simulink model "MSFartoystyringSCtuning"  (R2017b)
settings: Solver=ode45  StartTime=tstart  StopTime=tstop  RelTol=1e-3  EnableMultiTasking=on
values from neighbouring files (symbols this model uses):
  c = 1    [SCtune.m]
  p0 = zeros(2,1)    [SCtune.m]
  psi0 = 0    [SCtune.m]
  r0 = 0    [SCtune.m]
  tsamp = 10    [SCtune.m]
  v0 = [3 0]'    [SCtune.m]
undefined symbols (not defined in the file or in its folder): delta_max, heading_controller, K_iu, K_psi, K_pu, K_u, L_pp, msfartoystyring, n_max, speed_controller, T_psi, T_u
settings Model: ExtModeAutoUpdateStatusClock=off  Creator=christh  LastModifiedBy=sigtot
settings DataIOCC: LimitDataPoints=on  SaveFormat=Array  SignalLoggingSaveFormat=ModelDataLogs
settings OptimizationCC: ExpressionDepthLimit=2147483647  InitFltsAndDblsToZero=on  LifeSpan=inf
settings DebuggingCC: UnderspecifiedInitializationDetection=Classic  MergeDetectMultiDrivingBlocksExec=none  SolverPrmCheckMsg=warning  FcnCallInpInsideContextMsg=warning  StateNameClashWarn=warning  SFUnexpectedBacktrackingDiag=warning  SFNoUnconditionalDefaultTransitionDiag=warning
settings HardwareCC: ProdBitPerPointer=32  ProdBitPerSizeT=32  ProdBitPerPtrDiffT=32  ProdLargestAtomicFloat=None  ProdIntDivRoundTo=Undefined  ProdEndianess=Unspecified  ProdWordSize=32  ProdHWDeviceType=32-bit Generic
settings ModelReferenceCC: PropagateSignalLabelsOutOfModel=off
settings CodeAppCC: StateflowObjectComments=on
settings GRTTargetCC: TargetLangStandard=C89/C90 (ANSI)  GeneratePreprocessorConditionals=Disable all  CombineOutputUpdateFcns=off  GRTInterface=on
settings ConfigComp: CovMetricSettings=dw  CovHtmlReporting=on  CovSaveCumulativeToWorkspaceVar=on  CovSaveSingleToWorkspaceVar=on  CovExternalEMLEnable=off

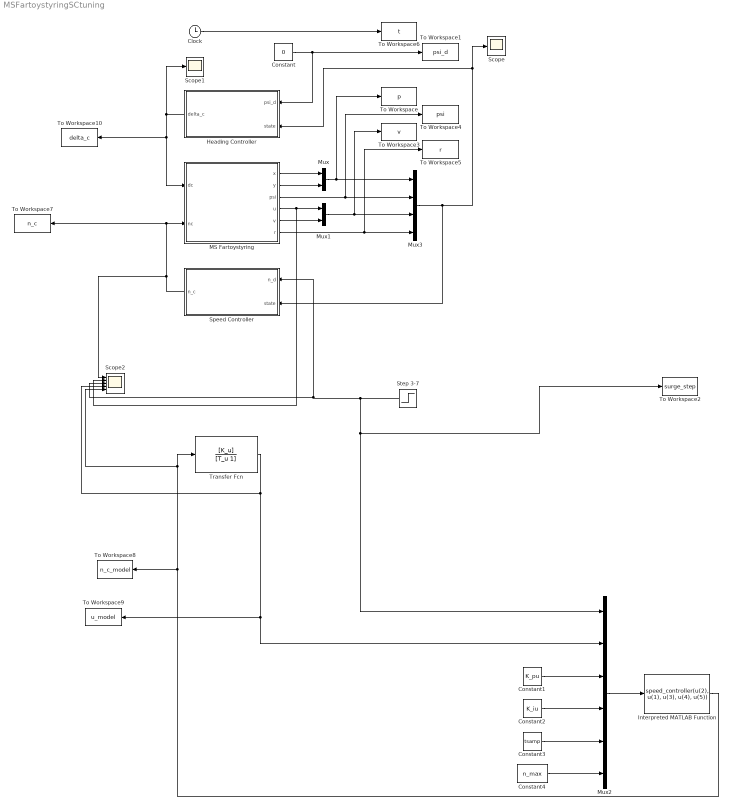
== system MSFartoystyringSCtuning ==
  Clock : Clock
  Constant : Constant  Value=0
  Constant1 : Constant  Value=K_pu
  Constant2 : Constant  Value=K_iu
  Constant3 : Constant  Value=tsamp
  Constant4 : Constant  Value=n_max
  "Heading Controller " : Subsystem
  Interpreted MATLAB Function : MATLABFcn  MATLABFcn=speed_controller(u(2), u(1), u(3), u(4), u(5))
  MS Fartoystyring : Subsystem  mask(MS Fartoystyring for Assignment 3 G&C){x0=p0(1), y0=p0(2), u0=v0(1), v0=v0(2), psi0=psi0, r0=r0, c=c}
      mask prompts: x0 "x(t0) (m)"; y0 "y(t0) (m)"; u0 "u(t0) (m/s)"; v0 "v(t0) (m/s)"; psi0 "psi(t0) (rad)"; r0 "r(t0) (rad/s)"; c "current (0 or 1)"
      mask help:
      | Block corresponding to Figure 1 in the assignment text. Gives the response of the ship.
      |
      | The design speed of MS Fartoystyring is u=8.23 m/s.
      |
      | Input:
      | dc: commanded rudder (rad), dmax=25*pi/180
      | nc: commanded shaft speed (rad/s), nmax=85*2*pi/60
      |
      | Output:
      | x: north pos (m)
      | y: east pos (m)
      | u: surge (m/s)
      | v: sway (m/s)
      | psi: heading (rad)
      | r: yaw (rad/s)
      mask Help: Comments, bugs and help requests can be directed to the TA. Email on course website.
  Mux : Mux  Inputs=2
  Mux1 : Mux  Inputs=2
  Mux2 : Mux  Inputs=6
  Mux3 : Mux
  Scope : Scope
  Scope1 : Scope
  Scope2 : Scope  NumInputPorts=5
  Speed Controller : Subsystem
  Step 3-7 : Step  Time=1250  Before=3  After=7  SampleTime=0
  To Workspace : ToWorkspace  VariableName=p  SampleTime=tsamp
  To Workspace1 : ToWorkspace  VariableName=psi_d  SampleTime=tsamp
  To Workspace10 : ToWorkspace  VariableName=delta_c  SampleTime=tsamp
  To Workspace2 : ToWorkspace  VariableName=surge_step  SampleTime=tsamp
  To Workspace3 : ToWorkspace  VariableName=v  SampleTime=tsamp
  To Workspace4 : ToWorkspace  VariableName=psi  SampleTime=tsamp
  To Workspace5 : ToWorkspace  VariableName=r  SampleTime=tsamp
  To Workspace6 : ToWorkspace  VariableName=t  SampleTime=tsamp
  To Workspace7 : ToWorkspace  VariableName=n_c  SampleTime=tsamp
  To Workspace8 : ToWorkspace  VariableName=n_c_model  SampleTime=tsamp
  To Workspace9 : ToWorkspace  VariableName=u_model  SampleTime=tsamp
  Transfer Fcn : TransferFcn  Numerator=[K_u]  Denominator=[T_u 1]
  wires:
  Clock/1 -> To Workspace6/1
  MS Fartoystyring/1(x) -> Mux/1
  MS Fartoystyring/2(y) -> Mux/2
  MS Fartoystyring/4(u) -> Scope2/2, Mux1/1
  MS Fartoystyring/5(v) -> Mux1/2
  Mux/1 -> To Workspace/1, Mux3/1
  Mux1/1 -> To Workspace3/1, Mux3/3
  MS Fartoystyring/3(psi) -> To Workspace4/1, Mux3/2
  MS Fartoystyring/6(r) -> To Workspace5/1, Mux3/4
  Mux3/1 -> Speed Controller/2(state), Scope/1, "Heading Controller "/2(state)
  "Heading Controller "/1(delta_c) -> To Workspace10/1, MS Fartoystyring/1(dc), Scope1/1
  Constant/1 -> "Heading Controller "/1(psi_d), To Workspace1/1
  Speed Controller/1(n_c) -> To Workspace7/1, MS Fartoystyring/2(nc), Scope2/1
  Constant2/1 -> Mux2/4
  Interpreted MATLAB Function/1 -> Scope2/5, Transfer Fcn/1, To Workspace8/1
  Mux2/1 -> Interpreted MATLAB Function/1
  Step 3-7/1 -> To Workspace2/1, Mux2/1, Speed Controller/1(n_d), Scope2/3
  Constant3/1 -> Mux2/5
  Constant4/1 -> Mux2/6
  Transfer Fcn/1 -> Scope2/4, To Workspace9/1, Mux2/2
  Constant1/1 -> Mux2/3

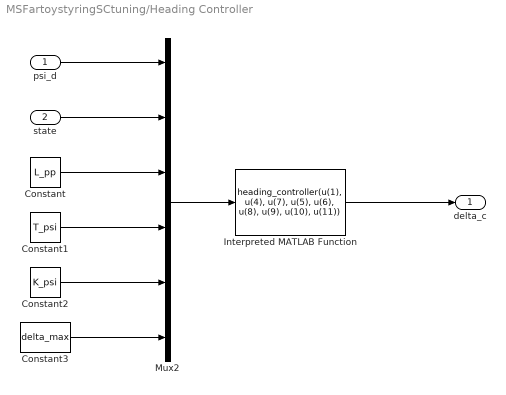
== system MSFartoystyringSCtuning/Heading Controller  ==
  psi_d : Inport
  state : Inport  Port=2
  Constant : Constant  Value=L_pp
  Constant1 : Constant  Value=T_psi
  Constant2 : Constant  Value=K_psi
  Constant3 : Constant  Value=delta_max
  Interpreted MATLAB Function : MATLABFcn  MATLABFcn=heading_controller(u(1), u(4), u(7), u(5), u(6), u(8), u(9), u(10), u(11))
  Mux2 : Mux  Inputs=6
  delta_c : Outport
  wires:
  Interpreted MATLAB Function/1 -> delta_c/1
  Mux2/1 -> Interpreted MATLAB Function/1
  psi_d/1 -> Mux2/1
  state/1 -> Mux2/2
  Constant/1 -> Mux2/3
  Constant1/1 -> Mux2/4
  Constant2/1 -> Mux2/5
  Constant3/1 -> Mux2/6

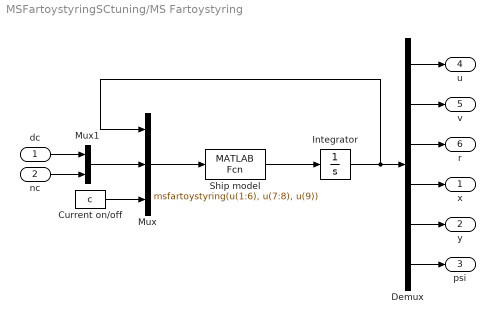
== system MSFartoystyringSCtuning/MS Fartoystyring ==
  dc : Inport
  nc : Inport  Port=2
  Current on/off : Constant  Value=c
  Demux : Demux  Outputs=6
  Integrator : Integrator  InitialCondition=[u0 v0 r0 x0 y0 psi0]'
  Mux : Mux  Inputs=3
  Mux1 : Mux  Inputs=2
  Ship model : MATLABFcn  MATLABFcn=msfartoystyring(u(1:6), u(7:8), u(9))  OutputDimensions=6
  x : Outport
  y : Outport  Port=2
  psi : Outport  Port=3
  u : Outport  Port=4
  v : Outport  Port=5
  r : Outport  Port=6
  wires:
  Integrator/1 -> Mux/1, Demux/1
  Mux1/1 -> Mux/2
  dc/1 -> Mux1/1
  nc/1 -> Mux1/2
  Demux/1 -> u/1
  Demux/2 -> v/1
  Demux/3 -> r/1
  Demux/4 -> x/1
  Demux/5 -> y/1
  Demux/6 -> psi/1
  Current on/off/1 -> Mux/3
  Ship model/1 -> Integrator/1
  Mux/1 -> Ship model/1

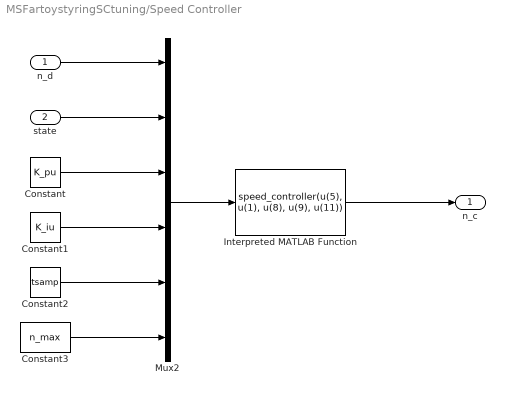
== system MSFartoystyringSCtuning/Speed Controller ==
  n_d : Inport
  state : Inport  Port=2
  Constant : Constant  Value=K_pu
  Constant1 : Constant  Value=K_iu
  Constant2 : Constant  Value=tsamp
  Constant3 : Constant  Value=n_max
  Interpreted MATLAB Function : MATLABFcn  MATLABFcn=speed_controller(u(5), u(1), u(8), u(9), u(11))
  Mux2 : Mux  Inputs=6
  n_c : Outport
  wires:
  Interpreted MATLAB Function/1 -> n_c/1
  Mux2/1 -> Interpreted MATLAB Function/1
  n_d/1 -> Mux2/1
  state/1 -> Mux2/2
  Constant/1 -> Mux2/3
  Constant1/1 -> Mux2/4
  Constant2/1 -> Mux2/5
  Constant3/1 -> Mux2/6
